simulink model "rl"  (R2023a)
settings: Solver=FixedStepAuto  StartTime=0.0  StopTime=100  FixedStep=0.002  RelTol=1e-3  EnableMultiTasking=on
values from neighbouring files (symbols this model uses):
  Inz = 1538    [MAIN.m]
  Iz = [5.12e6, 8.42,0, 8.42,0, 8.42,0, 8.42, 8.85, 1.62, 2.06, 0.0037,0.377]    [MAIN.m]
  Kx = zeros(n+1, n+1)    [MAIN.m]
  Kz = [K(2)      -K(2)    0         0         0         0    0 ... (first row only)    [MAIN.m]
  Mx = Mx + triu(Mx, 1)'    [MAIN.m]
  Mz = zeros(7,7)    [MAIN.m]
undefined symbols (not defined in the file or in its folder): Kd1, Kd2, Kp1, Kp2
libraries: slpidlib x2
settings Model: ExtModeTrigDuration=10000  Creator=AUSIM-ZJD  LastModifiedBy=AUSIM-ZJD
settings SolverCC: AlgebraicLoopSolver=TrustRegion  PositivePriorityOrder=on
settings DataIOCC: ReturnWorkspaceOutputs=off
settings OptimizationCC: LifeSpan=inf
settings DebuggingCC: UnconnectedInputMsg=warning  UnconnectedOutputMsg=warning  UnconnectedLineMsg=warning  ArithmeticOperatorsInVariantConditions=warning
settings ModelReferenceCC: EnableRefExpFcnMdlSchedulingChecks=on
settings SFSimCC: SimUseLocalCustomCode=off  CustomCodeUndefinedFunction=UseInterfaceOnly
settings RTWCC: Description=QUARC Win64 Target  SystemTargetFile=quarc_win64.tlc  TemplateMakefile=quarc_default_tmf  RTWUseLocalCustomCode=off
settings CodeAppCC: StateflowObjectComments=on
settings STFCustomTargetCC: TargetPreCompLibLocation=C:\PROGRA~3\QUARC\lib\2016a\win64\release  UseToolchainInfoCompliant=off  SystemTargetFile=quarc_win64.tlc
settings GRTTargetCC: TargetPreCompLibLocation=C:\PROGRA~3\QUARC\lib\2016a\win64\release  ParMdlRefBuildCompliant=off  CompOptLevelCompliant=off  CombineOutputUpdateFcns=off  MatFileLogging=off  CPPClassGenCompliant=off  GRTInterface=on  UseToolchainInfoCompliant=off  ExtMode=on  ExtModeMexFile=quarc_comm
settings ConfigComp: CovMetricSettings=dswe

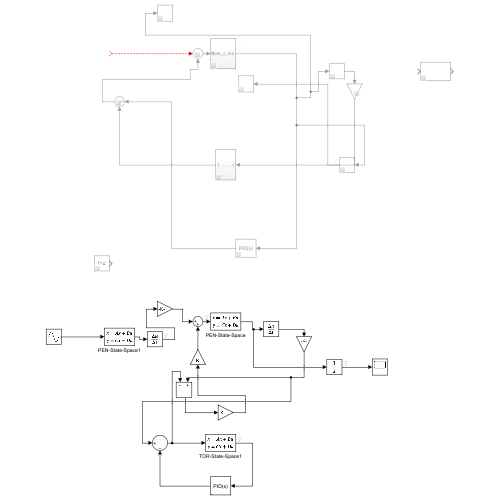
[thumbnail: Simulink's stored preview of the top-level diagram]
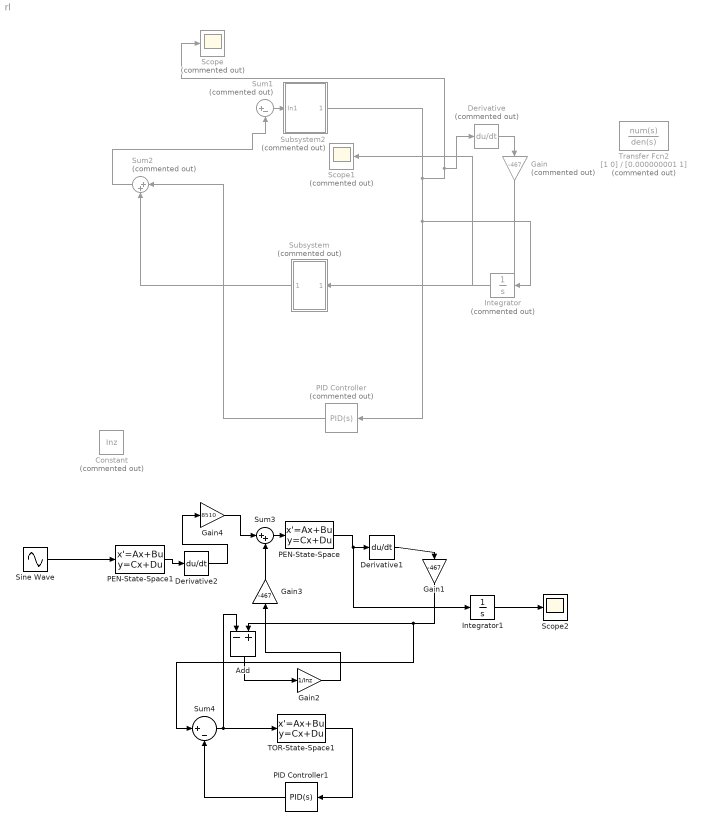
== system rl ==
  Add : Sum  Inputs=-+
  Constant : Constant  Commented=on  Value=Inz
  Derivative : Derivative  Commented=on
  Derivative1 : Derivative
  Derivative2 : Derivative
  Gain : Gain  Commented=on  Gain=-467
  Gain1 : Gain  Gain=-467
  Gain2 : Gain  Gain=1/Inz
  Gain3 : Gain  Gain=-467
  Gain4 : Gain  Gain=8510
  Integrator : Integrator  Commented=on
  Integrator1 : Integrator
  PEN-State-Space : StateSpace  A=[zeros(12, 12), eye(12); -Mx\Kx, zeros(12, 12)]  B=[zeros(12, 1); Mx\ [0; 0; 0; 0; 0; 0;0; 0; 0; 0; 0; 1]]  C=[ 0, 0, 0, 0, 0,0,0, 0, 0, 0, 0, 0, 0, 0, 0, 0, 0,0,0, 0, 0, 0, 0, 1]  D=0  InitialCondition=[0, 0, 0, 0, 0,0, 0,0, 0, 0, 0, 0, 0,0,0,0, 0,0, 0, 0, 0, 0, 0,0]
  PEN-State-Space1 : StateSpace  A=[zeros(12, 12), eye(12); -Mx\Kx, zeros(12, 12)]  B=[zeros(12, 1); Mx\ [1; 0; 0; 0; 0; 0;0; 0; 0; 0; 0; 0]]  C=[ 0, 0, 0, 0, 0,0,0, 0, 0, 0, 0, 0, 0, 0, 0, 0, 0,0,0, 0, 0, 0, 0, 1]  D=0  InitialCondition=[0, 0, 0, 0, 0,0, 0,0, 0, 0, 0, 0, 0,0,0,0, 0,0, 0, 0, 0, 0, 0,0]
  PID Controller : slpidlib/PID Controller  Commented=on  Controller=PID  Form=Parallel  TimeDomain=Continuous-time  UseExternalTs=off  SampleTime=-1  IntegratorMethod=Forward Euler  FilterMethod=Forward Euler  ControllerParametersSource=internal  P=76  I=0  UseKiTs=off  D=0  N=100  UseFilter=on  TunerSelectOption=Transfer Function Based (PID Tuner App)  InitialConditionSource=internal  InitialConditionForIntegrator=0  InitialConditionForFilter=0  DifferentiatorICPrevScaledInput=0  ExternalReset=none  TrackingMode=off  Kt=1  LimitOutput=off  SatLimitsSource=internal  UpperSaturationLimit=inf  LowerSaturationLimit=-inf  LinearizeAsGain=on  AntiWindupMode=none  Kb=1  LimitIntegrator=off  UpperIntegratorSaturationLimit=inf  LowerIntegratorSaturationLimit=-inf  POutMin=[]  POutMax=[]  IOutMin=[]  IOutMax=[]  DOutMin=[]  DOutMax=[]  NOutMin=[]  NOutMax=[]  SumOutMin=[]  SumOutMax=[]  SaturationOutMin=[]  SaturationOutMax=[]  PParamMin=[]  PParamMax=[]  IParamMin=[]  IParamMax=[]  DParamMin=[]  DParamMax=[]  NParamMin=[]  NParamMax=[]  KbParamMin=[]  KbParamMax=[]  KtParamMin=[]  KtParamMax=[]  KbOutMin=[]  KbOutMax=[]  KtOutMin=[]  KtOutMax=[]  IntegratorOutMin=[]  IntegratorOutMax=[]  FilterOutMin=[]  FilterOutMax=[]  SumI1OutMin=[]  SumI1OutMax=[]  SumI2OutMin=[]  SumI2OutMax=[]  SumI3OutMin=[]  SumI3OutMax=[]  SumI4OutMin=[]  SumI4OutMax=[]  SumDOutMin=[]  SumDOutMax=[]  DifferentiatorOutMin=[]  DifferentiatorOutMax=[]  FilterDiffOutCoefMin=[]  FilterDiffOutCoefMax=[]  ReciprocalOutMin=[]  ReciprocalOutMax=[]  SumDenOutMin=[]  SumDenOutMax=[]  SumNumOutMin=[]  SumNumOutMax=[]  DivideOutMin=[]  DivideOutMax=[]  UdiffTsProdOutMin=[]  UdiffTsProdOutMax=[]  NTsProdOutMin=[]  NTsProdOutMax=[]  UintegralTsProdOutMin=[]  UintegralTsProdOutMax=[]  UngainTsProdOutMin=[]  UngainTsProdOutMax=[]  ClampingZeroOutDataTypeStr=Inherit: Inherit via back propagation  ClampingZeroOutMin=[]  ClampingZeroOutMax=[]  FilterDenConstantOutDataTypeStr=Inherit: Inherit via back propagation  FilterDenConstantOutMin=[]  FilterDenConstantOutMax=[]  PCopyOutDataTypeStr=Inherit: Inherit via back propagation  PCopyOutMin=[]  PCopyOutMax=[]  NCopyOutDataTypeStr=Inherit: Inherit via back propagation  NCopyOutMin=[]  NCopyOutMax=[]  IntegratorContinuousStateAttributes=''  IntegratorStateMustResolveToSignalObject=off  IntegratorRTWStateStorageClass=Auto  FilterContinuousStateAttributes=''  FilterStateMustResolveToSignalObject=off  FilterRTWStateStorageClass=Auto  ParallelPVariant=InternalParameters  IdealPVariant=Disabled  IVariant=InternalParameters  DVariant=InternalParameters  IntegratorVariant=Continuous  SatVariant=Disabled  AWVariant=Passthrough  PCopyVariant=Disabled  TRVariant=Disabled  FdbkBlocksVariant=Forward  IdealPFdbkVariant=Disabled  SatFdbkVariant=Disabled  DerivativeFilterVariant=ContFilter  NVariant=InternalParameters  NCopyVariant=Disabled  FilterICVariant=InternalICsFilter  IntegratorICVariant=InternalICs  ExternalResetVariant=Disabled  TRSumVariant=Passthrough  SumFdbkVariant=Disabled  SumVariant=Sum_PID  TsampFilterVariant=InternalTs  TsampNgainVariant=Passthrough  TsampIntegralVariant=Disabled_SignalSpec  ExternalSaturationOutDataTypeStr=Inherit: Same as second input
  PID Controller1 : slpidlib/PID Controller  Controller=PID  Form=Parallel  TimeDomain=Continuous-time  UseExternalTs=off  SampleTime=-1  IntegratorMethod=Forward Euler  FilterMethod=Forward Euler  ControllerParametersSource=internal  P=76  I=0  UseKiTs=off  D=0  N=100  UseFilter=on  TunerSelectOption=Transfer Function Based (PID Tuner App)  InitialConditionSource=internal  InitialConditionForIntegrator=0  InitialConditionForFilter=0  DifferentiatorICPrevScaledInput=0  ExternalReset=none  TrackingMode=off  Kt=1  LimitOutput=off  SatLimitsSource=internal  UpperSaturationLimit=inf  LowerSaturationLimit=-inf  LinearizeAsGain=on  AntiWindupMode=none  Kb=1  LimitIntegrator=off  UpperIntegratorSaturationLimit=inf  LowerIntegratorSaturationLimit=-inf  POutMin=[]  POutMax=[]  IOutMin=[]  IOutMax=[]  DOutMin=[]  DOutMax=[]  NOutMin=[]  NOutMax=[]  SumOutMin=[]  SumOutMax=[]  SaturationOutMin=[]  SaturationOutMax=[]  PParamMin=[]  PParamMax=[]  IParamMin=[]  IParamMax=[]  DParamMin=[]  DParamMax=[]  NParamMin=[]  NParamMax=[]  KbParamMin=[]  KbParamMax=[]  KtParamMin=[]  KtParamMax=[]  KbOutMin=[]  KbOutMax=[]  KtOutMin=[]  KtOutMax=[]  IntegratorOutMin=[]  IntegratorOutMax=[]  FilterOutMin=[]  FilterOutMax=[]  SumI1OutMin=[]  SumI1OutMax=[]  SumI2OutMin=[]  SumI2OutMax=[]  SumI3OutMin=[]  SumI3OutMax=[]  SumI4OutMin=[]  SumI4OutMax=[]  SumDOutMin=[]  SumDOutMax=[]  DifferentiatorOutMin=[]  DifferentiatorOutMax=[]  FilterDiffOutCoefMin=[]  FilterDiffOutCoefMax=[]  ReciprocalOutMin=[]  ReciprocalOutMax=[]  SumDenOutMin=[]  SumDenOutMax=[]  SumNumOutMin=[]  SumNumOutMax=[]  DivideOutMin=[]  DivideOutMax=[]  UdiffTsProdOutMin=[]  UdiffTsProdOutMax=[]  NTsProdOutMin=[]  NTsProdOutMax=[]  UintegralTsProdOutMin=[]  UintegralTsProdOutMax=[]  UngainTsProdOutMin=[]  UngainTsProdOutMax=[]  ClampingZeroOutDataTypeStr=Inherit: Inherit via back propagation  ClampingZeroOutMin=[]  ClampingZeroOutMax=[]  FilterDenConstantOutDataTypeStr=Inherit: Inherit via back propagation  FilterDenConstantOutMin=[]  FilterDenConstantOutMax=[]  PCopyOutDataTypeStr=Inherit: Inherit via back propagation  PCopyOutMin=[]  PCopyOutMax=[]  NCopyOutDataTypeStr=Inherit: Inherit via back propagation  NCopyOutMin=[]  NCopyOutMax=[]  IntegratorContinuousStateAttributes=''  IntegratorStateMustResolveToSignalObject=off  IntegratorRTWStateStorageClass=Auto  FilterContinuousStateAttributes=''  FilterStateMustResolveToSignalObject=off  FilterRTWStateStorageClass=Auto  ParallelPVariant=InternalParameters  IdealPVariant=Disabled  IVariant=InternalParameters  DVariant=InternalParameters  IntegratorVariant=Continuous  SatVariant=Disabled  AWVariant=Passthrough  PCopyVariant=Disabled  TRVariant=Disabled  FdbkBlocksVariant=Forward  IdealPFdbkVariant=Disabled  SatFdbkVariant=Disabled  DerivativeFilterVariant=ContFilter  NVariant=InternalParameters  NCopyVariant=Disabled  FilterICVariant=InternalICsFilter  IntegratorICVariant=InternalICs  ExternalResetVariant=Disabled  TRSumVariant=Passthrough  SumFdbkVariant=Disabled  SumVariant=Sum_PID  TsampFilterVariant=InternalTs  TsampNgainVariant=Passthrough  TsampIntegralVariant=Disabled_SignalSpec  ExternalSaturationOutDataTypeStr=Inherit: Same as second input
  Scope : Scope  Commented=on
  Scope1 : Scope  Commented=on
  Scope2 : Scope
  Sine Wave : Sin  Amplitude=5000  SampleTime=0
  Subsystem : Subsystem  Commented=on
  Subsystem2 : Subsystem  Commented=on
  Sum1 : Sum  Commented=on  Inputs=|+-
  Sum2 : Sum  Commented=on  Inputs=|++
  Sum3 : Sum  Inputs=|++
  Sum4 : Sum  Inputs=|+-
  TOR-State-Space1 : StateSpace  A=[zeros(7, 7), eye(7); -inv(Mz)*Kz, zeros(7, 7)]  B=[zeros(7, 1); inv(Mz) * [0; 0; 0; 0; 0; 0;1]]  C=[0, 0, 0, 0, 0, 0,0,0, 0, 0, 0, 0, 0, 1]  D=0  InitialCondition=[0, 0, 0, 0, 0,0, 0,0, 0, 0, 0, 0, 0,0]
  Transfer Fcn2 : TransferFcn  Commented=on  Numerator=[1 0]  Denominator=[0.000000001 1]
  wires:
  Subsystem2/1(theta_x_dot) -> Integrator/1, PID Controller/1, Scope/1, Derivative/1
  Sum1/1 -> Subsystem2/1(In1)
  Gain/1 -> Subsystem/1(In1)
  PID Controller/1 -> Sum2/1
  Integrator/1 -> Scope1/1
  Derivative/1 -> Gain/1
  Sum2/1 -> Sum1/2
  Subsystem/1(Out1) -> Sum2/2
  ? -> Sum1/1
  PEN-State-Space/1 -> Integrator1/1, Derivative1/1
  Derivative1/1 -> Gain1/1
  Gain1/1 -> Sum4/1, Add/2
  Add/1 -> Gain2/1
  Gain2/1 -> Gain3/1
  Sum3/1 -> PEN-State-Space/1
  Gain3/1 -> Sum3/2
  TOR-State-Space1/1 -> PID Controller1/1
  PID Controller1/1 -> Sum4/2
  Sum4/1 -> TOR-State-Space1/1, Add/1
  Sine Wave/1 -> PEN-State-Space1/1
  Integrator1/1 -> Scope2/1
  PEN-State-Space1/1 -> Derivative2/1
  Derivative2/1 -> Gain4/1
  Gain4/1 -> Sum3/1

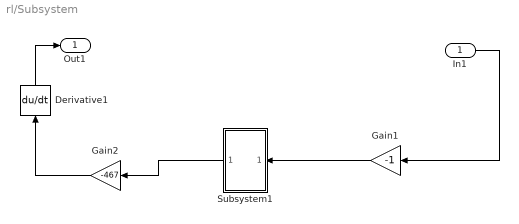
== system rl/Subsystem ==
  In1 : Inport
  Derivative1 : Derivative
  Gain1 : Gain  Gain=-1
  Gain2 : Gain  Gain=-467
  Subsystem1 : Subsystem
  Out1 : Outport
  wires:
  Gain2/1 -> Derivative1/1
  Gain1/1 -> Subsystem1/1(In1)
  Subsystem1/1(theta_z_dot) -> Gain2/1
  Derivative1/1 -> Out1/1
  In1/1 -> Gain1/1

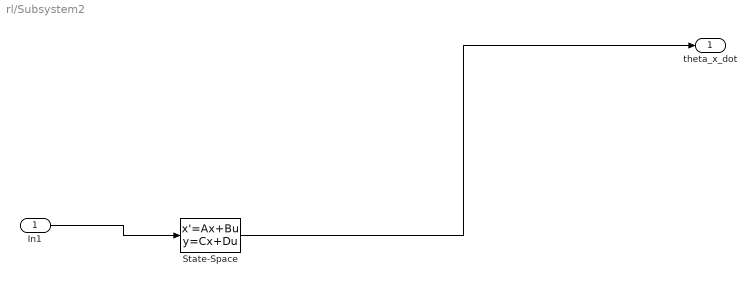
== system rl/Subsystem2 ==
  In1 : Inport
  State-Space : StateSpace  A=[zeros(12, 12), eye(12); -Mx\Kx, zeros(12, 12)]  B=[zeros(12, 1); Mx\ [0; 0; 0; 0; 0; 0;0; 0; 0; 0; 0; 1]]  C=[ 0, 0, 0, 0, 0,0,0, 0, 0, 0, 0, 0, 0, 0, 0, 0, 0,0,0, 0, 0, 0, 0, 1]  D=0  InitialCondition=[0, 0, 0, 0, 0,0, 0,0, 0, 0, 0, 0, 0,0,0,0, 0,0, 0, 0, 0, 0, 0,0]
  theta_x_dot : Outport
  wires:
  In1/1 -> State-Space/1
  State-Space/1 -> theta_x_dot/1

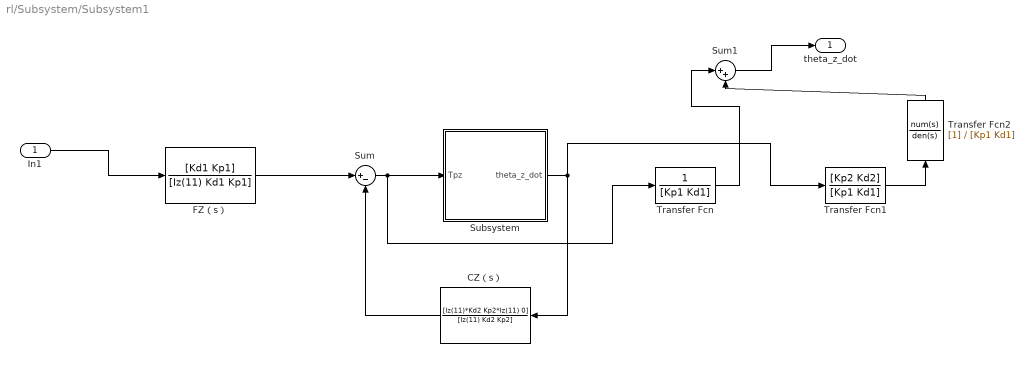
== system rl/Subsystem/Subsystem1 ==
  In1 : Inport
  CZ（s） : TransferFcn  Numerator=[Iz(11)*Kd2 Kp2*Iz(11) 0]  Denominator=[Iz(11) Kd2 Kp2]
  FZ（s） : TransferFcn  Numerator=[Kd1 Kp1]  Denominator=[Iz(11) Kd1 Kp1]
  Subsystem : Subsystem
  Sum : Sum  Inputs=|+-
  Sum1 : Sum  Inputs=|++
  Transfer Fcn : TransferFcn  Denominator=[Kp1 Kd1]
  Transfer Fcn1 : TransferFcn  Numerator=[Kp2 Kd2]  Denominator=[Kp1 Kd1]
  Transfer Fcn2 : TransferFcn  Denominator=[Kp1 Kd1]
  theta_z_dot : Outport
  wires:
  CZ（s）/1 -> Sum/2
  FZ（s）/1 -> Sum/1
  In1/1 -> FZ（s）/1
  Sum/1 -> Transfer Fcn/1, Subsystem/1(Tpz)
  Subsystem/1(theta_z_dot) -> Transfer Fcn1/1, CZ（s）/1
  Transfer Fcn/1 -> Sum1/1
  Transfer Fcn1/1 -> Transfer Fcn2/1
  Transfer Fcn2/1 -> Sum1/2
  Sum1/1 -> theta_z_dot/1

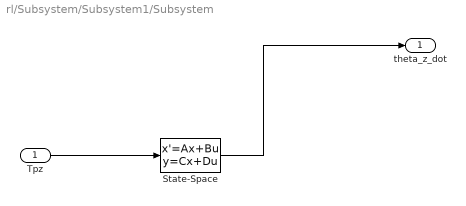
== system rl/Subsystem/Subsystem1/Subsystem ==
  Tpz : Inport
  State-Space : StateSpace  A=[zeros(7, 7), eye(7); -inv(Mz)*Kz, zeros(7, 7)]  B=[zeros(7, 1); inv(Mz) * [0; 0; 0; 0; 0; 0;1]]  C=[0, 0, 0, 0, 0, 0,0,0, 0, 0, 0, 0, 0, 1]  D=0  InitialCondition=[0, 0, 0, 0, 0,0, 0,0, 0, 0, 0, 0, 0,0]
  theta_z_dot : Outport
  wires:
  State-Space/1 -> theta_z_dot/1
  Tpz/1 -> State-Space/1
